simulink model "case2_bottomtank"  (R2015b)
settings: Solver=FixedStepAuto  StartTime=0  StopTime=40.65  FixedStep=0.05  RelTol=1e-3
values from neighbouring files (symbols this model uses):
  AdBottom = (pi*(0.01)^2)/4    (= 7.85398163397e-05)    [case1.m]    (also in case1_val.m; case2.m; case2_val.m; case3.m)
  AreaBottom = (pi*(0.08)^2)/4    (= 0.00502654824574)    [case1.m]    (also in case1_val.m; case2.m; case2_val.m; case3.m)
  Cd2 = b2(i)    [case2.m]    (also in case2_val.m = 0.45)
  g = 9.81    [case1.m]    (also in case1_val.m; case2.m; case2_val.m; case3.m)
settings Model: Creator=guilh_000  LastModifiedBy=guilh_000

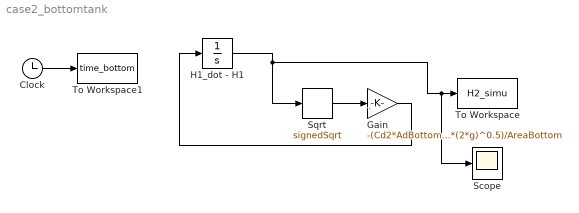
== system case2_bottomtank ==
  note: `
  Clock : Clock
  Gain : Gain  Gain=-(Cd2*AdBottom*(2*g)^0.5)/AreaBottom
  H1_dot - H1 : Integrator  InitialCondition=(3.98E+01)*0.01
  Scope : Scope
  Sqrt : Sqrt  Operator=signedSqrt  SaturateOnIntegerOverflow=on
  To Workspace : ToWorkspace  VariableName=H2_simu  SampleTime=-1
  To Workspace1 : ToWorkspace  VariableName=time_bottom  SampleTime=-1
  wires:
  H1_dot - H1/1 -> Scope/1, To Workspace/1, Sqrt/1
  Sqrt/1 -> Gain/1
  Gain/1 -> H1_dot - H1/1
  Clock/1 -> To Workspace1/1
